simulink model "LLC"  (R2024b)
settings: Solver=ode4  StartTime=0.0  StopTime=0.1  FixedStep=1/(1000*1000*12)  RelTol=1e-3
libraries: spsSeriesRLCBranchLib x6, spsVoltageMeasurementLib x6, spsCurrentMeasurementLib x5, spsDiodeLib x4, spsMosfetLib x2, spsDCVoltageSourceLib x1, spsLinearTransformerLib x1, spspowerguiLib x1
settings Model: Creator=adity  LastModifiedBy=adity

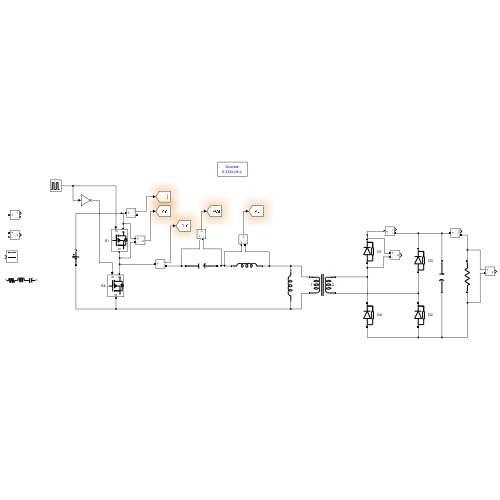
[thumbnail: Simulink's stored preview of the top-level diagram]
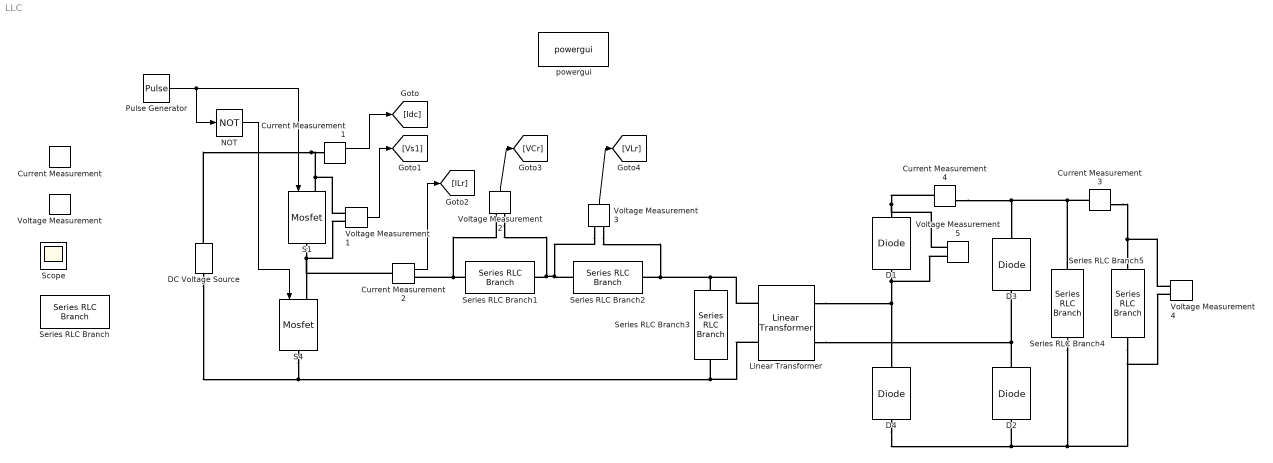
== system LLC ==
  Current Measurement{,1..4} (5 alike) : spsCurrentMeasurementLib/Current Measurement  PhasorSimulation=off  OutputType=Complex  PSBequivalent=0
  D{1..4} (4 alike) : spsDiodeLib/Diode  Ron=1e-2  Lon=0  Vf=0  IC=0  UseSnubber=0  Rs=500  Cs=250e-9  Measurements=off
  DC Voltage Source : spsDCVoltageSourceLib/DC Voltage Source  Amplitude=60  Measurements=None
  Linear Transformer : spsLinearTransformerLib/Linear Transformer  UNITS=SI  NominalPower=[ 250e6 50 ]  winding1=[7.35e+05*5 4.3218*25 0.55027*25]  winding2=[3.15e+05 0.7938 0.10107]  ThreeWindings=off  winding3=[3.15e+05 0.7938 0.10107]  RmLm=[1.0804e+06 3439.2]  Measurements=None  DataType=on
  NOT : Logic  Operator=NOT  IconShape=distinctive  AllPortsSameDT=off  OutDataTypeStr=boolean
  Pulse Generator : DiscretePulseGenerator  PulseType=Time based  Period=1/(12e3)  PulseWidth=50
  S1 : spsMosfetLib/Mosfet  Ron=1e-2  Lon=0  Rd=1e-2  Vfd=0  IC=0  Rs=1e5  Cs=inf  Measurements=off
  S4 : spsMosfetLib/Mosfet  Ron=1e-2  Lon=0  Rd=1e-2  Vfd=0  IC=0  Rs=1e5  Cs=inf  Measurements=off
  Scope : Scope
  Series RLC Branch : spsSeriesRLCBranchLib/Series RLC Branch  LConnTagsString=__new0  RConnTagsString=__new0  BranchType=RLC  Resistance=1  Inductance=1e-3  SetiL0=off  InitialCurrent=0  Capacitance=1e-6  Setx0=off  InitialVoltage=0  Measurements=None
  Series RLC Branch1 : spsSeriesRLCBranchLib/Series RLC Branch  LConnTagsString=__new0  RConnTagsString=__new0  BranchType=C  Resistance=1  Inductance=1e-3  SetiL0=off  InitialCurrent=0  Capacitance=90e-9  Setx0=off  InitialVoltage=0  Measurements=None
  Series RLC Branch2 : spsSeriesRLCBranchLib/Series RLC Branch  LConnTagsString=__new0  RConnTagsString=__new0  BranchType=L  Resistance=1  Inductance=800e-6  SetiL0=off  InitialCurrent=0  Capacitance=7e-9  Setx0=off  InitialVoltage=0  Measurements=Branch voltage and current
  Series RLC Branch3 : spsSeriesRLCBranchLib/Series RLC Branch  LConnTagsString=__new0  RConnTagsString=__new0  BranchType=L  Resistance=1  Inductance=3779.45e-6  SetiL0=off  InitialCurrent=0  Capacitance=7e-9  Setx0=off  InitialVoltage=0  Measurements=None
  Series RLC Branch4 : spsSeriesRLCBranchLib/Series RLC Branch  LConnTagsString=__new0  RConnTagsString=__new0  BranchType=C  Resistance=1  Inductance=1e-3  SetiL0=off  InitialCurrent=0  Capacitance=420e-6  Setx0=off  InitialVoltage=0  Measurements=None
  Series RLC Branch5 : spsSeriesRLCBranchLib/Series RLC Branch  LConnTagsString=__new0  RConnTagsString=__new0  BranchType=R  Resistance=2  Inductance=1e-3  SetiL0=off  InitialCurrent=0  Capacitance=7e-9  Setx0=off  InitialVoltage=0  Measurements=None
  Voltage Measurement{,1..5} (6 alike) : spsVoltageMeasurementLib/Voltage Measurement  PhasorSimulation=off  OutputType=Complex  PSBequivalent=0
  powergui : spspowerguiLib/powergui  Priority=1  SimulationMode=Discrete  SampleTime=1/(1000*1000*12)  frequency=60  Iterations=50  frequencyindice=0  Pbase=100e6  ErrMax=1e-4  UnitsV=kV  UnitsW=MW  buscounter=0  FunctionMessages=off  echomessages=off  EnableUseOfTLC=off  CurrentSourceSwitches=off  DisableSnubberDevices=off  DisableRonSwitches=off  DisableVfSwitches=off  DisplayEquations=off  AutomaticDiscreteSolvers=off  SolverType=Tustin/Backward Euler (TBE)  Interpol=off  ExternalGateDelay=off  methode=off  Ts=100  x0status=blocks  SPID=on  SwTol=0  HookPort=off  NonlinearTolerance=1e-4  nMaxIteration=100  ContinueOnMaxIteration=off  RestoreLinks=warning  ResistiveCurrentMeasurement=off  Frange=[0:2:500]  Ylog=off  Xlog=on  ShowGrid=off  save=off  variable=ZData  structure=0  ZoomFFT=off  StartTime=0.0  cycles=1  DisplayStyle=1  fundamental=60  FreqAxis=off  MaxFrequency=1000  frequencyindicesteady=1  RmsSteady=1  display=off
  wires:
  Pulse Generator/1 -> NOT/1, S1/1
  NOT/1 -> S4/1
  Current Measurement1/1 -> [Idc]
  Voltage Measurement1/1 -> [Vs1]
  Current Measurement2/1 -> [ILr]
  Voltage Measurement2/1 -> [VCr]
  Voltage Measurement3/1 -> [VLr]
  connections:
  S1/RConn1 -- S4/LConn1 -- Current Measurement2/LConn1 -- Voltage Measurement1/LConn2
  S4/RConn1 -- Linear Transformer/LConn2 -- Series RLC Branch3/RConn1 -- DC Voltage Source/LConn1
  S1/LConn1 -- DC Voltage Source/RConn1 -- Current Measurement1/LConn1 -- Voltage Measurement1/LConn1
  Series RLC Branch2/LConn1 -- Voltage Measurement2/LConn2 -- Series RLC Branch1/RConn1 -- Voltage Measurement3/LConn1
  Series RLC Branch3/LConn1 -- Linear Transformer/LConn1 -- Voltage Measurement3/LConn2 -- Series RLC Branch2/RConn1
  Series RLC Branch1/LConn1 -- Voltage Measurement2/LConn1 -- Current Measurement2/RConn1
  D2/RConn1 -- Linear Transformer/RConn2 -- D3/LConn1
  Series RLC Branch4/LConn1 -- Current Measurement3/LConn1 -- Current Measurement4/RConn1 -- D3/RConn1
  D1/LConn1 -- Voltage Measurement5/LConn2 -- Linear Transformer/RConn1 -- D4/RConn1
  D4/LConn1 -- D2/LConn1 -- Series RLC Branch4/RConn1 -- Voltage Measurement4/LConn2 -- Series RLC Branch5/RConn1
  Current Measurement3/RConn1 -- Voltage Measurement4/LConn1 -- Series RLC Branch5/LConn1
  Current Measurement4/LConn1 -- Voltage Measurement5/LConn1 -- D1/RConn1
